simulink model "RobotModel1"  (R2025b)
settings: Solver=VariableStepAuto  StartTime=0.0  StopTime=40  RelTol=1e-3  AbsTol=1e-3  EnableMultiTasking=on
undefined symbols (not defined in the file): waypoints, X, Y, Z
libraries: sm_lib x57, nesl_utility x33, slpidlib x2, robotalgslib x1, sharedtransform x1
(part 3 of 3)

== matlab function RobotModel1/Subsystem1/MATLAB Function ==
  data: lock_en input; tau output; q input; dq input
function tau = JointSoftLock(lock_en, q, dq)
%#codegen
% lock_en: 0/1 (double 或 uint8 均可)

Kp = 1200.0;  Kd = 20.0;  tau_lim = 300.0;

% 统一成 uint8(0/1)
u8 = uint8(lock_en ~= 0);

persistent q_hold last_en
if isempty(q_hold),  q_hold  = q;          end      % double
if isempty(last_en), last_en = uint8(0);   end      % uint8

% 上升沿：0 -> 1
if (last_en == uint8(0)) && (u8 ~= uint8(0))
    q_hold = q;
end
last_en = u8;

if u8 ~= 0
    q_ref = q_hold; dq_ref = 0.0;
    tau = Kp*(q_ref - q) + Kd*(dq_ref - dq);
else
    tau = 0.0;
end

% 限幅
tau = max(min(tau, tau_lim), -tau_lim);

== matlab function RobotModel1/Subsystem2/MATLAB Function ==
  data: lock_en input; tau output; q input; dq input
function tau = JointSoftLock(lock_en, q, dq)
%#codegen
% lock_en: 0/1 (double 或 uint8 均可)

Kp = 1200.0;  Kd = 20.0;  tau_lim = 300.0;

% 统一成 uint8(0/1)
u8 = uint8(lock_en ~= 0);

persistent q_hold last_en
if isempty(q_hold),  q_hold  = q;          end      % double
if isempty(last_en), last_en = uint8(0);   end      % uint8

% 上升沿：0 -> 1
if (last_en == uint8(0)) && (u8 ~= uint8(0))
    q_hold = q;
end
last_en = u8;

if u8 ~= 0
    q_ref = q_hold; dq_ref = 0.0;
    tau = Kp*(q_ref - q) + Kd*(dq_ref - dq);
else
    tau = 0.0;
end

% 限幅
tau = max(min(tau, tau_lim), -tau_lim);

== matlab function RobotModel1/Subsystem2/MATLAB Function1 ==
  data: lock_en input; tau output; q input; dq input
function tau = JointSoftLock(lock_en, q, dq)
%#codegen
% lock_en: 0/1 (double 或 uint8 均可)

Kp = 1200.0;  Kd = 20.0;  tau_lim = 300.0;

% 统一成 uint8(0/1)
u8 = uint8(lock_en ~= 0);

persistent q_hold last_en
if isempty(q_hold),  q_hold  = q;          end      % double
if isempty(last_en), last_en = uint8(0);   end      % uint8

% 上升沿：0 -> 1
if (last_en == uint8(0)) && (u8 ~= uint8(0))
    q_hold = q;
end
last_en = u8;

if u8 ~= 0
    q_ref = q_hold; dq_ref = 0.0;
    tau = Kp*(q_ref - q) + Kd*(dq_ref - dq);
else
    tau = 0.0;
end

% 限幅
tau = max(min(tau, tau_lim), -tau_lim);

== matlab function RobotModel1/Subsystem3/MATLAB Function ==
  data: lock_en input; tau output; q input; dq input
function tau = JointSoftLock(lock_en, q, dq)
%#codegen
% lock_en: 0/1 (double 或 uint8 均可)

Kp = 1200.0;  Kd = 20.0;  tau_lim = 300.0;

% 统一成 uint8(0/1)
u8 = uint8(lock_en ~= 0);

persistent q_hold last_en
if isempty(q_hold),  q_hold  = q;          end      % double
if isempty(last_en), last_en = uint8(0);   end      % uint8

% 上升沿：0 -> 1
if (last_en == uint8(0)) && (u8 ~= uint8(0))
    q_hold = q;
end
last_en = u8;

if u8 ~= 0
    q_ref = q_hold; dq_ref = 0.0;
    tau = Kp*(q_ref - q) + Kd*(dq_ref - dq);
else
    tau = 0.0;
end

% 限幅
tau = max(min(tau, tau_lim), -tau_lim);

== matlab function RobotModel1/Subsystem3/MATLAB Function1 ==
  data: lock_en input; tau output; q input; dq input
function tau = JointSoftLock(lock_en, q, dq)
%#codegen
% lock_en: 0/1 (double 或 uint8 均可)

Kp = 1200.0;  Kd = 20.0;  tau_lim = 300.0;

% 统一成 uint8(0/1)
u8 = uint8(lock_en ~= 0);

persistent q_hold last_en
if isempty(q_hold),  q_hold  = q;          end      % double
if isempty(last_en), last_en = uint8(0);   end      % uint8

% 上升沿：0 -> 1
if (last_en == uint8(0)) && (u8 ~= uint8(0))
    q_hold = q;
end
last_en = u8;

if u8 ~= 0
    q_ref = q_hold; dq_ref = 0.0;
    tau = Kp*(q_ref - q) + Kd*(dq_ref - dq);
else
    tau = 0.0;
end

% 限幅
tau = max(min(tau, tau_lim), -tau_lim);

== matlab function RobotModel1/Subsystem4/MATLAB Function ==
  data: lock_en input; tau output; q input; dq input
function tau = JointSoftLock(lock_en, q, dq)
%#codegen
% lock_en: 0/1 (double 或 uint8 均可)

Kp = 1200.0;  Kd = 20.0;  tau_lim = 300.0;

% 统一成 uint8(0/1)
u8 = uint8(lock_en ~= 0);

persistent q_hold last_en
if isempty(q_hold),  q_hold  = q;          end      % double
if isempty(last_en), last_en = uint8(0);   end      % uint8

% 上升沿：0 -> 1
if (last_en == uint8(0)) && (u8 ~= uint8(0))
    q_hold = q;
end
last_en = u8;

if u8 ~= 0
    q_ref = q_hold; dq_ref = 0.0;
    tau = Kp*(q_ref - q) + Kd*(dq_ref - dq);
else
    tau = 0.0;
end

% 限幅
tau = max(min(tau, tau_lim), -tau_lim);

== matlab function RobotModel1/Subsystem4/MATLAB Function1 ==
  data: lock_en input; tau output; q input; dq input
function tau = JointSoftLock(lock_en, q, dq)
%#codegen
% lock_en: 0/1 (double 或 uint8 均可)

Kp = 1200.0;  Kd = 20.0;  tau_lim = 300.0;

% 统一成 uint8(0/1)
u8 = uint8(lock_en ~= 0);

persistent q_hold last_en
if isempty(q_hold),  q_hold  = q;          end      % double
if isempty(last_en), last_en = uint8(0);   end      % uint8

% 上升沿：0 -> 1
if (last_en == uint8(0)) && (u8 ~= uint8(0))
    q_hold = q;
end
last_en = u8;

if u8 ~= 0
    q_ref = q_hold; dq_ref = 0.0;
    tau = Kp*(q_ref - q) + Kd*(dq_ref - dq);
else
    tau = 0.0;
end

% 限幅
tau = max(min(tau, tau_lim), -tau_lim);

== matlab function RobotModel1/MATLAB Function ==
  data: v input; delta output; w input; L input; v output
function [delta, v] = Diff2Ackermann(v, w, L)
% input: 
%   v - Linear velocity (m/s)
%   w - Angular velocity (rad/s)
%   L -  (m)
%
% output:
%   delta - front whell ratation angel (rad)
%   v     -  velocity(m/s)
if abs(v) < 1e-3
    delta = 0;
else
    delta = atan(L * w / v);   % pure pursuit function
end

== matlab function RobotModel1/MATLAB Function1 ==
  data: v input; wL_cmd output; w input; T input; r input; wR_cmd output
function [wL_cmd, wR_cmd] = wheelSpeedCmd(v, w, T, r)
% v: 线速度 [m/s]
% w: 航向角速度 [rad/s]
% T: 后轮距 [m]
% r: 车轮半径 [m]

vL = v - 0.5*T*w;
vR = v + 0.5*T*w;

wL_cmd = vL / r;
wR_cmd = vR / r;
end
